simulink model "fl"  (R2015a)
settings: Solver=ode45  StartTime=0.0  StopTime=10.0  RelTol=1e-3
settings Model: Creator=BML  LastModifiedBy=BML

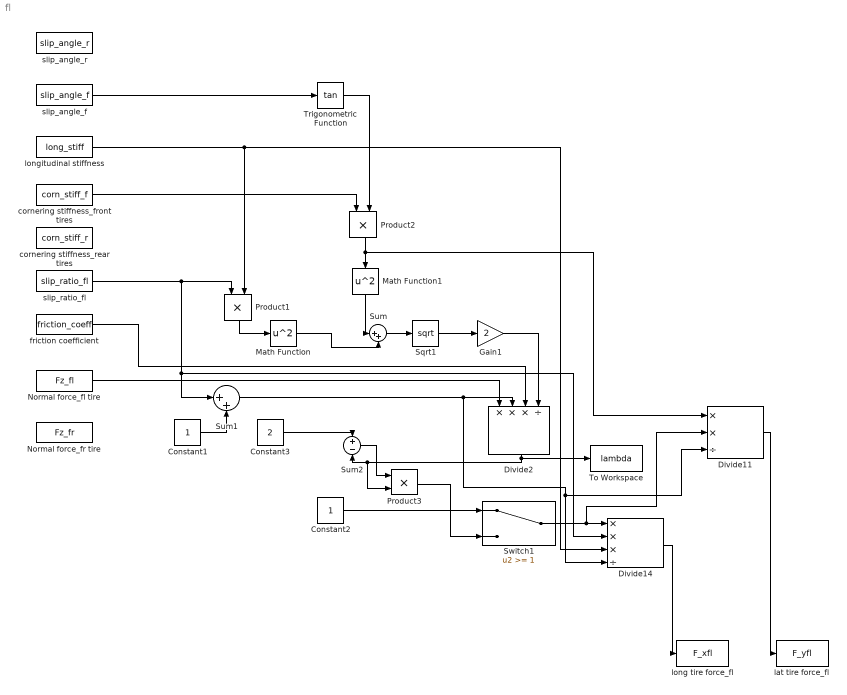
== system fl ==
  Constant1 : Constant
  Constant2 : Constant
  Constant3 : Constant  Value=2
  Divide11 : Product  Inputs=**/
  Divide14 : Product  Inputs=***/
  Divide2 : Product  Inputs=***/
  Gain1 : Gain  Gain=2
  Math Function : Math  Operator=square  SaturateOnIntegerOverflow=on
  Math Function1 : Math  Operator=square  SaturateOnIntegerOverflow=on
  Normal force_fl tire : FromWorkspace  VariableName=Fz_fl  SampleTime=0
  Normal force_fr tire : FromWorkspace  VariableName=Fz_fr  SampleTime=0
  Product1 : Product
  Product2 : Product
  Product3 : Product
  Sqrt1 : Sqrt  SaturateOnIntegerOverflow=on
  Sum : Sum  Inputs=|++
  Sum1 : Sum  Inputs=|++
  Sum2 : Sum  Inputs=+-
  Switch1 : Switch  Threshold=1
  To Workspace : ToWorkspace  VariableName=lambda  SaveFormat=Timeseries  SampleTime=-1
  Trigonometric Function : Trigonometry  Operator=tan
  cornering stiffness_front tires : FromWorkspace  VariableName=corn_stiff_f  SampleTime=0
  cornering stiffness_rear tires : FromWorkspace  VariableName=corn_stiff_r  SampleTime=0
  friction coefficient : FromWorkspace  VariableName=friction_coeff  SampleTime=0
  lat tire force_fl : ToWorkspace  VariableName=F_yfl  SaveFormat=Timeseries  SampleTime=-1
  long tire force_fl : ToWorkspace  VariableName=F_xfl  SaveFormat=Timeseries  SampleTime=-1
  longitudinal stiffness : FromWorkspace  VariableName=long_stiff  SampleTime=0
  slip_angle_f : FromWorkspace  VariableName=slip_angle_f  SampleTime=0
  slip_angle_r : FromWorkspace  VariableName=slip_angle_r  SampleTime=0
  slip_ratio_fl : FromWorkspace  VariableName=slip_ratio_fl  SampleTime=0
  wires:
  Product1/1 -> Math Function/1
  slip_angle_f/1 -> Trigonometric Function/1
  Trigonometric Function/1 -> Product2/2
  Product2/1 -> Divide11/1, Math Function1/1
  Math Function1/1 -> Sum/1
  Math Function/1 -> Sum/2
  Sum/1 -> Sqrt1/1
  Sqrt1/1 -> Gain1/1
  Constant1/1 -> Sum1/2
  slip_ratio_fl/1 -> Divide14/2, Sum1/1, Product1/1
  Gain1/1 -> Divide2/4
  Normal force_fl tire/1 -> Divide2/1
  friction coefficient/1 -> Divide2/3
  Constant2/1 -> Switch1/1
  Constant3/1 -> Sum2/1
  Sum2/1 -> Product3/1
  Divide2/1 -> Product3/2, Sum2/2, To Workspace/1
  Product3/1 -> Switch1/3
  Sum1/1 -> Divide11/3, Divide14/4, Divide2/2
  longitudinal stiffness/1 -> Product1/2, Divide14/3
  Divide14/1 -> long tire force_fl/1
  cornering stiffness_front tires/1 -> Product2/1
  Switch1/1 -> Divide11/2, Divide14/1
  Divide11/1 -> lat tire force_fl/1
